simulink model "Motor"  (R2023a)
settings: Solver=VariableStepAuto  StartTime=0.0  StopTime=10.0  RelTol=1e-3
settings Model: Creator=Waffle  LastModifiedBy=Waffle

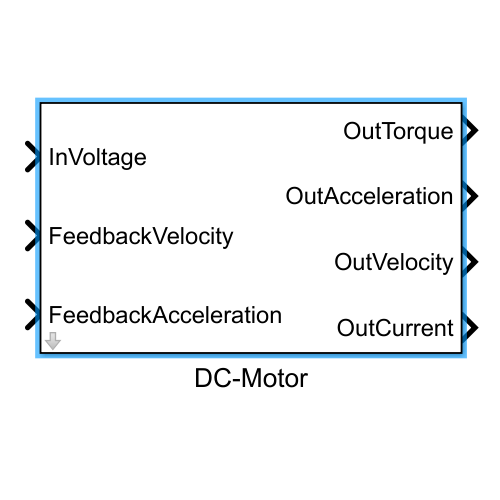
[thumbnail: Simulink's stored preview of the top-level diagram]
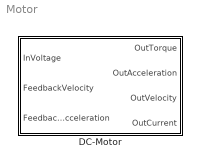
== system Motor ==
  DC-Motor : Subsystem  mask{R=10, L=0.000350, kw=10, km=0.016, J_motor=0.0000005, vis_friction_coef_motor=0.5}
      mask prompts: R "Активное сопротивление якоря, Ом"; L "Индуктивность якоря, Гн"; kw "Коэф. скорости двигателя, об/сек"; km "Коэф. момента двигателя, Н*м/А"; J_motor "Момент инерции, кг*м^2"; vis_friction_coef_motor "Коэф. вязкого трения двигателя"

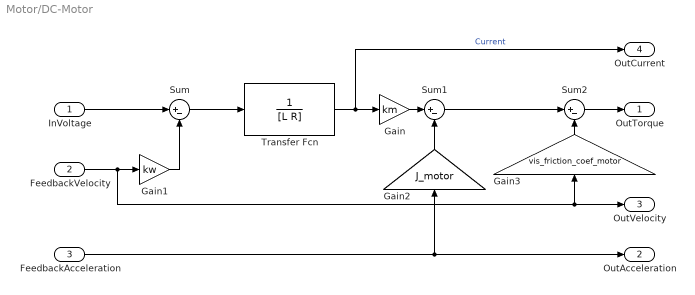
== system Motor/DC-Motor ==
  InVoltage : Inport
  FeedbackVelocity : Inport  Port=2
  FeedbackAcceleration : Inport  Port=3
  Gain : Gain  Gain=km
  Gain1 : Gain  Gain=kw
  Gain2 : Gain  Gain=J_motor
  Gain3 : Gain  Gain=vis_friction_coef_motor
  Sum : Sum  Inputs=|+-
  Sum1 : Sum  Inputs=|+-
  Sum2 : Sum  Inputs=|+-
  Transfer Fcn : TransferFcn  Denominator=[L R]
  OutTorque : Outport
  OutAcceleration : Outport  Port=2
  OutVelocity : Outport  Port=3
  OutCurrent : Outport  Port=4
  wires:
  InVoltage/1 -> Sum/1
  Sum/1 -> Transfer Fcn/1
  Transfer Fcn/1 -> OutCurrent/1, Gain/1  "Current"
  FeedbackVelocity/1 -> OutVelocity/1, Gain3/1, Gain1/1
  Gain1/1 -> Sum/2
  FeedbackAcceleration/1 -> OutAcceleration/1, Gain2/1
  Gain/1 -> Sum1/1
  Gain2/1 -> Sum1/2
  Sum1/1 -> Sum2/1
  Sum2/1 -> OutTorque/1
  Gain3/1 -> Sum2/2
